simulink model "Simulation"  (R2025b)
settings: Solver=ode5  StartTime=0.0  StopTime=10.0  FixedStep=.005  RelTol=1e-3
values from neighbouring files (symbols this model uses):
  A = model.a    [param_control.m]
  B = model.b    [param_control.m]
  C = model.c    [param_control.m]
  D = model.d    [param_control.m]
  H = 1/ (C_cmd*((eye(4) - A + B*K)\B))    [param_control.m]
  K = place(A, B, z_p)    [param_control.m]
  L = place(A',C', z_po)'    [param_control.m]
  nx = 4    [ident_model.m]    (also in param_control.m)
settings Model: Creator=Bako  LastModifiedBy=victor

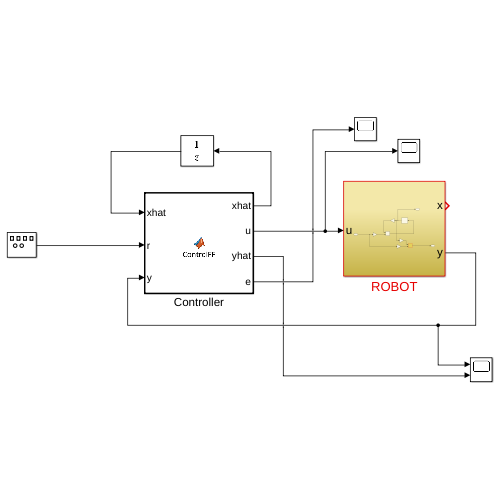
[thumbnail: Simulink's stored preview of the top-level diagram]
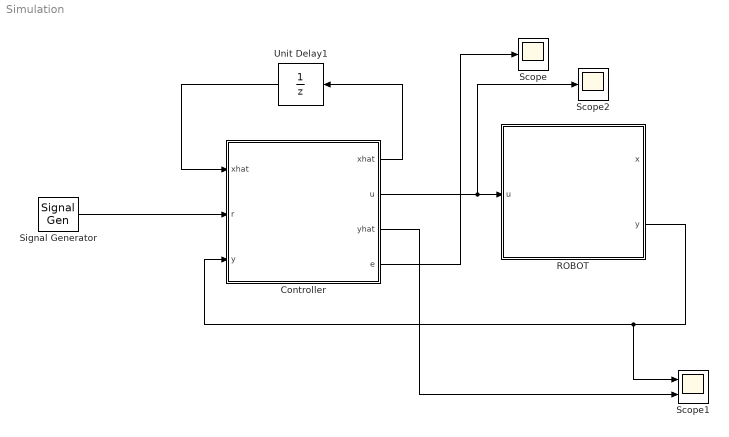
== system Simulation ==
  Controller : MATLAB Function  TreatAsAtomicUnit=on
  ROBOT : Subsystem
  Scope : Scope
      settings: ActiveDisplayYMinimum=-68.703939718571988  ActiveDisplayYMaximum=118.33545746714789
  Scope1 : Scope  NumInputPorts=2
      settings: ActiveDisplayYMinimum=-55.837166635500857  ActiveDisplayYMaximum=6.21932223374876
  Scope2 : Scope
      settings: ActiveDisplayYMinimum=-1  ActiveDisplayYMaximum=1  DataLoggingVariableName=ScopeData2
  Signal Generator : SignalGenerator  WaveForm=square  Amplitude=50  Frequency=.05
  Unit Delay1 : UnitDelay  InitialCondition=zeros(nx,1)  SampleTime=-1  HasFrameUpgradeWarning=on
  wires:
  Controller/1(xhat) -> Unit Delay1/1
  Unit Delay1/1 -> Controller/1("xhat ")
  Controller/2(u) -> Scope2/1, ROBOT/1(u)
  ROBOT/2(y) -> Scope1/1, Controller/3(y)
  Controller/4(e) -> Scope/1
  Controller/3(yhat) -> Scope1/2
  Signal Generator/1 -> Controller/2(r)

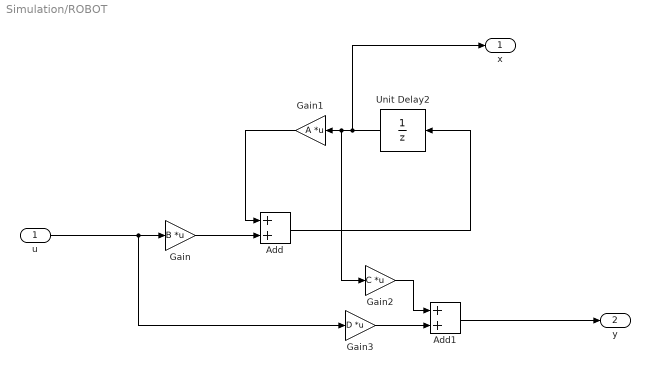
== system Simulation/ROBOT ==
  u : Inport
  Add : Sum
  Add1 : Sum
  Gain : Gain  Gain=B  Multiplication=Matrix(K*u) (u vector)
  Gain1 : Gain  Gain=A  Multiplication=Matrix(K*u) (u vector)
  Gain2 : Gain  Gain=C  Multiplication=Matrix(K*u) (u vector)
  Gain3 : Gain  Gain=D  Multiplication=Matrix(K*u) (u vector)
  Unit Delay2 : UnitDelay  InitialCondition=zeros(nx,1)  SampleTime=-1  HasFrameUpgradeWarning=on
  x : Outport
  y : Outport  Port=2
  wires:
  u/1 -> Gain3/1, Gain/1
  Gain/1 -> Add/2
  Unit Delay2/1 -> x/1, Gain2/1, Gain1/1
  Gain1/1 -> Add/1
  Add/1 -> Unit Delay2/1
  Add1/1 -> y/1
  Gain2/1 -> Add1/1
  Gain3/1 -> Add1/2

== matlab function Simulation/Controller ==
  data: xhat output; xhat input; r input; u output; y input; A parameter; B parameter; C parameter; D parameter; L parameter; K parameter; yhat output; e output; H parameter
function [xhat,u,yhat,e] = ControlFF(xhat,r,y,A,B,C,D,L,K, H)

z = y(1);
e = r-z;
u = -K*xhat+H*r; 

yhat = C*xhat+D*u;
xhat = A*xhat+B*u+L*(y-yhat);
